simulink model "linear_inverted_pendulum_tracking_controller_simplified"  (Simulink 7.9)
settings: Solver=ode3  StartTime=0.0  StopTime=7.7  FixedStep=1/100  RelTol=1e-3
values from neighbouring files (symbols this model uses):
  f = 200    [WPG_results.m]    (also in WPG_results_10.m = wpg_param.frequency; WPG_results_2.m = wpg_param.frequency; WPG_results_3.m = wpg_param.frequency; WPG_results_4.m = wpg_param.frequency)
  k1 = -q(1)*q(2)-1    [WPG_results.m]    (also in WPG_results_10.m; WPG_results_2.m; WPG_results_3.m; WPG_results_4.m)
  k2 = (q(1)+q(2))/-q(3)    [WPG_results.m]    (also in WPG_results_10.m; WPG_results_2.m; WPG_results_3.m; WPG_results_4.m)
  k3 = w    [WPG_results.m]    (also in WPG_results_10.m; WPG_results_2.m; WPG_results_3.m; WPG_results_4.m)
  sx_d = [time sx_d]    [WPG_results.m]    (also in WPG_sim.m; control_layer_zmp_com_init.m = [time sx_d_y]; control_layer_zmp_com_init_2.m = [time sx_d_x])
  w = wpg_param.w    [WPG_results.m]    (also in WPG_results_10.m; WPG_results_2.m; WPG_results_3.m; WPG_results_4.m)
  x_d = [time x_d]    [WPG_results.m]    (also in WPG_sim.m; control_layer_zmp_com_init.m = [time x_d_y]; control_layer_zmp_com_init_2.m = [time x_d_x])
libraries: commnoisgen2 x1
settings Model: Creator=pajon  LastModifiedBy=pajon

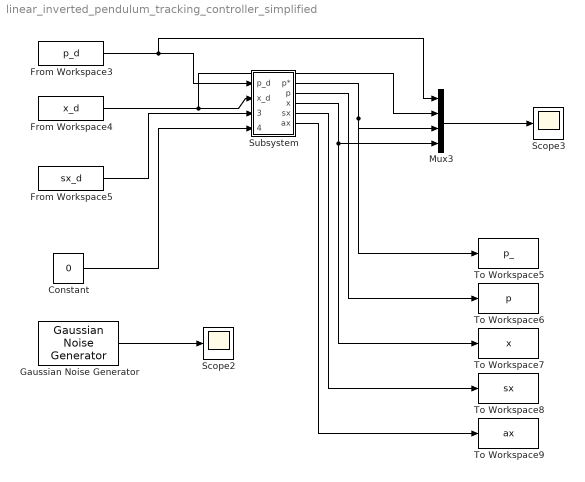
== system linear_inverted_pendulum_tracking_controller_simplified ==
  Constant : Constant  Value=0
  From Workspace3 : FromWorkspace  VariableName=p_d  SampleTime=0
  From Workspace4 : FromWorkspace  VariableName=x_d  SampleTime=0
  From Workspace5 : FromWorkspace  VariableName=sx_d  SampleTime=0
  Gaussian Noise Generator : commnoisgen2/Gaussian Noise Generator  m=0  d=0.001/6  s=41  Ts=1/f  frameBased=off  sampPerFrame=1  orient=off  outDataType=double
  Mux3 : Mux
  Scope2 : Scope
      settings: SaveName=ScopeData2
  Scope3 : Scope
      settings: TimeRange=15
  Subsystem : Subsystem
  To Workspace5 : ToWorkspace  VariableName=p_  SampleTime=-1
  To Workspace6 : ToWorkspace  VariableName=p  SampleTime=-1
  To Workspace7 : ToWorkspace  VariableName=x  SampleTime=-1
  To Workspace8 : ToWorkspace  VariableName=sx  SampleTime=-1
  To Workspace9 : ToWorkspace  VariableName=ax  SampleTime=-1
  wires:
  From Workspace3/1 -> Subsystem/1(p_d), Mux3/1
  From Workspace4/1 -> Subsystem/2(x_d), Mux3/2
  From Workspace5/1 -> Subsystem/3(sx_d)
  Mux3/1 -> Scope3/1
  Gaussian Noise Generator/1 -> Scope2/1
  Subsystem/1(p*) -> Mux3/3, To Workspace5/1
  Subsystem/2(p) -> To Workspace6/1
  Subsystem/3(x) -> Mux3/4, To Workspace7/1
  Subsystem/4(sx) -> To Workspace8/1
  Subsystem/5(ax) -> To Workspace9/1
  Constant/1 -> Subsystem/4(perturb)

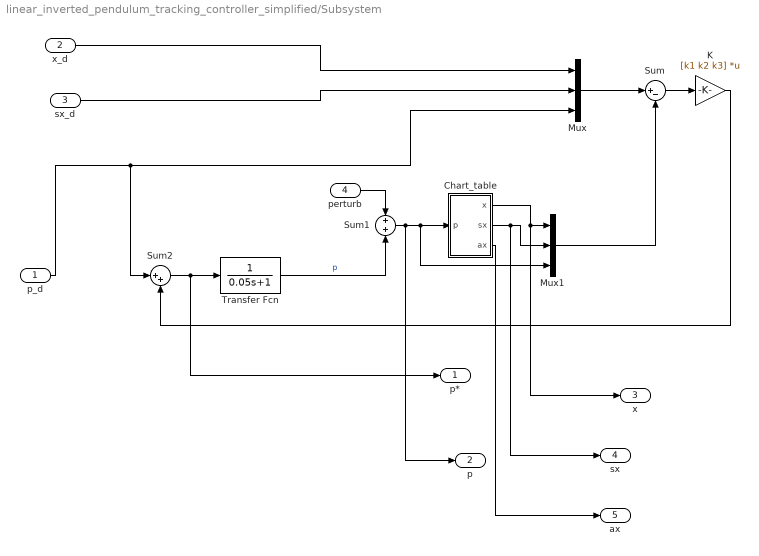
== system linear_inverted_pendulum_tracking_controller_simplified/Subsystem ==
  p_d : Inport
  x_d : Inport  Port=2
  sx_d : Inport  Port=3
  perturb : Inport  Port=4
  Chart_table : Subsystem
  K : Gain  Gain=[k1 k2 k3]  Multiplication=Matrix(K*u)
  Mux : Mux  Inputs=3
  Mux1 : Mux  Inputs=3
  Sum : Sum  Inputs=|+-
  Sum1 : Sum
  Sum2 : Sum  Inputs=|++
  Transfer Fcn : TransferFcn  Denominator=[0.05 1]
  p* : Outport
  p : Outport  Port=2
  x : Outport  Port=3
  sx : Outport  Port=4
  ax : Outport  Port=5
  wires:
  Sum1/1 -> Chart_table/1(p), Mux1/3, p/1
  Mux/1 -> Sum/1
  Mux1/1 -> Sum/2
  Sum/1 -> K/1
  K/1 -> Sum2/2
  Sum2/1 -> Transfer Fcn/1, p*/1
  Transfer Fcn/1 -> Sum1/2  "p"
  Chart_table/1(x) -> Mux1/1, x/1
  Chart_table/2(sx) -> Mux1/2, sx/1
  p_d/1 -> Mux/3, Sum2/1
  perturb/1 -> Sum1/1
  Chart_table/3(ax) -> ax/1
  x_d/1 -> Mux/1
  sx_d/1 -> Mux/2

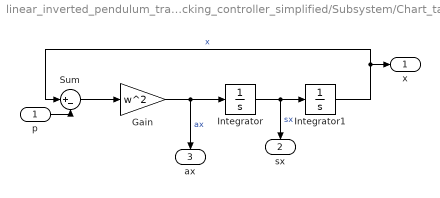
== system linear_inverted_pendulum_tracking_controller_simplified/Subsystem/Chart_table ==
  p : Inport
  Gain : Gain  Gain=w^2
  Integrator : Integrator  InitialCondition=sx_d(1,2)
  Integrator1 : Integrator  InitialCondition=x_d(1,2)
  Sum : Sum  Inputs=|+-
  x : Outport
  sx : Outport  Port=2
  ax : Outport  Port=3
  wires:
  Integrator/1 -> Integrator1/1, sx/1  "sx"
  Integrator1/1 -> Sum/1, x/1  "x"
  Gain/1 -> Integrator/1, ax/1  "ax"
  Sum/1 -> Gain/1
  p/1 -> Sum/2
